simulink model "ECM_Final"  (R2015b)
settings: Solver=ode1  StartTime=Tstart  StopTime=Tend  FixedStep=1  RelTol=1e-3
undefined symbols (not defined in the file): C1_values, capacity_points, dt, initialSoC, ocv_points, R0_values, R1_values, soc_points, SOC_values, temp_battery, Temp_values, temperature_points
libraries: simulink x1
settings Model: Creator=BJ  LastModifiedBy=aallam
settings DataIOCC: SaveFormat=Array  SignalLoggingSaveFormat=ModelDataLogs
settings OptimizationCC: ExpressionDepthLimit=2147483647
settings DebuggingCC: UnderspecifiedInitializationDetection=Classic  MergeDetectMultiDrivingBlocksExec=none  SolverPrmCheckMsg=warning  FcnCallInpInsideContextMsg=EnableAllAsWarning  StateNameClashWarn=warning
settings HardwareCC: ProdBitPerPointer=32  ProdLargestAtomicFloat=None  ProdIntDivRoundTo=Undefined  ProdEndianess=Unspecified  ProdWordSize=32  ProdHWDeviceType=32-bit Generic
settings GRTTargetCC: GeneratePreprocessorConditionals=Disable all
settings ConfigComp: CovModelRefEnable=Off

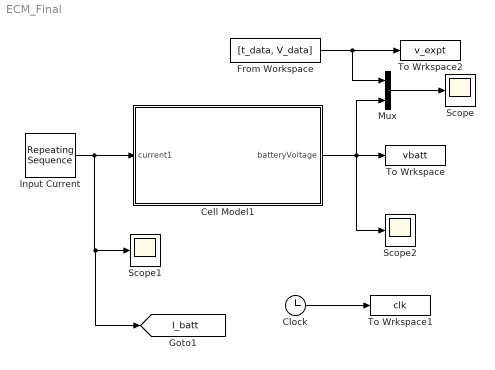
== system ECM_Final ==
  Cell Model1 : Subsystem
  Clock : Clock
  From Workspace : FromWorkspace  VariableName=[t_data, V_data]  SampleTime=0
  Input Current : simulink/Sources/Repeating Sequence  rep_seq_t=t_data  rep_seq_y=I_data
  Mux : Mux  Inputs=2
  Scope : Scope
  Scope1 : Scope
  Scope2 : Scope
  To Wrkspace : ToWorkspace  VariableName=vbatt  SampleTime=-1
  To Wrkspace1 : ToWorkspace  VariableName=clk  SampleTime=-1
  To Wrkspace2 : ToWorkspace  VariableName=v_expt  SampleTime=-1
  tag scope: I_batt=global
  wires:
  Cell Model1/1(batteryVoltage) -> Scope2/1, Mux/2, To Wrkspace/1
  Clock/1 -> To Wrkspace1/1
  From Workspace/1 -> Mux/1, To Wrkspace2/1
  Mux/1 -> Scope/1
  Input Current/1 -> [I_batt], Scope1/1, Cell Model1/1(current1)

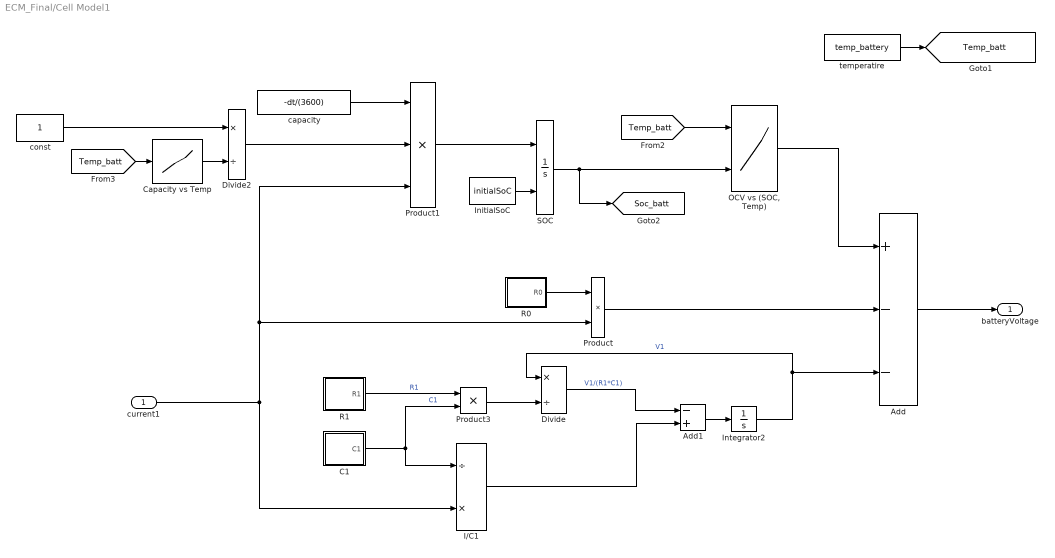
== system ECM_Final/Cell Model1 ==
  current1 : Inport
  Add : Sum  Inputs=+--
  Add1 : Sum  Inputs=-+
  C1 : Subsystem
  Capacity vs Temp : Lookup_n-D  NumberOfTableDimensions=1  BreakpointsForDimension1=temperature_points  BreakpointsForDimension2=soc_points  Table=capacity_points  RndMeth=Simplest  InputSameDT=on
  Divide : Product  Inputs=*/
  Divide2 : Product  Inputs=*/
  I/C1 : Product  Inputs=/*
  InitialSoC : Constant  Value=initialSoC
  Integrator2 : Integrator
  "OCV vs (SOC, Temp)" : Lookup_n-D  BreakpointsForDimension1=temperature_points  BreakpointsForDimension2=soc_points  Table=ocv_points  RndMeth=Simplest  InputSameDT=on
  Product : Product  RndMeth=Zero
  Product1 : Product  Inputs=3  RndMeth=Zero
  Product3 : Product  RndMeth=Zero
  R0 : Subsystem
  R1 : Subsystem
  SOC : Integrator  InitialConditionSource=external  InitialCondition=1
  capacity : Constant  Value=-dt/(3600)
  const : Constant
  temperatire : Constant  Value=temp_battery
  batteryVoltage : Outport
  tag scope: Soc_batt=global, Temp_batt=global
  wires:
  SOC/1 -> "OCV vs (SOC, Temp)"/2, [Soc_batt]
  Product1/1 -> SOC/1
  capacity/1 -> Product1/1
  Product/1 -> Add/2
  "OCV vs (SOC, Temp)"/1 -> Add/1
  Capacity vs Temp/1 -> Divide2/2
  InitialSoC/1 -> SOC/2
  R1/1(R1) -> Product3/1  "R1"
  C1/1(C1) -> Product3/2, I/C1/1  "C1"
  Integrator2/1 -> Add/3, Divide/1  "V1"
  I/C1/1 -> Add1/2
  Divide/1 -> Add1/1  "V1/(R1*C1)"
  Add1/1 -> Integrator2/1
  current1/1 -> Product1/3, Product/2, I/C1/2
  Add/1 -> batteryVoltage/1
  [Temp_batt] -> "OCV vs (SOC, Temp)"/1
  const/1 -> Divide2/1
  R0/1(R0) -> Product/1
  [Temp_batt] -> Capacity vs Temp/1
  Divide2/1 -> Product1/2
  Product3/1 -> Divide/2
  temperatire/1 -> [Temp_batt]

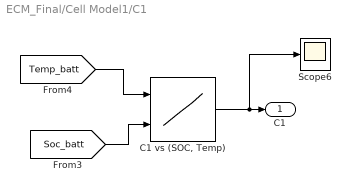
== system ECM_Final/Cell Model1/C1 ==
  "C1 vs (SOC, Temp)" : Lookup_n-D  BreakpointsForDimension1=Temp_values  BreakpointsForDimension2=SOC_values  Table=C1_values  InternalRulePriority=Speed  RndMeth=Simplest  InputSameDT=on
  Scope6 : Scope
  C1 : Outport
  wires:
  "C1 vs (SOC, Temp)"/1 -> Scope6/1, C1/1
  [Soc_batt] -> "C1 vs (SOC, Temp)"/2
  [Temp_batt] -> "C1 vs (SOC, Temp)"/1

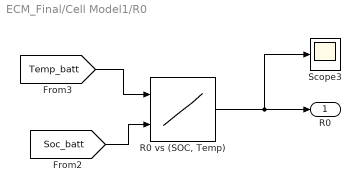
== system ECM_Final/Cell Model1/R0 ==
  "R0 vs (SOC, Temp)" : Lookup_n-D  BreakpointsForDimension1=Temp_values  BreakpointsForDimension2=SOC_values  Table=R0_values  InternalRulePriority=Speed  RndMeth=Simplest  InputSameDT=on
  Scope3 : Scope
  R0 : Outport
  wires:
  "R0 vs (SOC, Temp)"/1 -> Scope3/1, R0/1
  [Soc_batt] -> "R0 vs (SOC, Temp)"/2
  [Temp_batt] -> "R0 vs (SOC, Temp)"/1

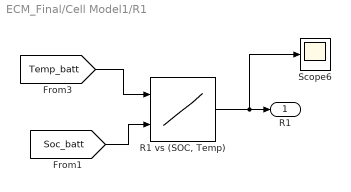
== system ECM_Final/Cell Model1/R1 ==
  "R1 vs (SOC, Temp)" : Lookup_n-D  BreakpointsForDimension1=Temp_values  BreakpointsForDimension2=SOC_values  Table=R1_values  InternalRulePriority=Speed  RndMeth=Simplest  InputSameDT=on
  Scope6 : Scope
  R1 : Outport
  wires:
  "R1 vs (SOC, Temp)"/1 -> Scope6/1, R1/1
  [Soc_batt] -> "R1 vs (SOC, Temp)"/2
  [Temp_batt] -> "R1 vs (SOC, Temp)"/1
